simulink model "PID"  (R2021a)
settings: Solver=FixedStepAuto  StartTime=0.0  StopTime=1  FixedStep=0.01  MaxStep=1  RelTol=1e-3
settings Model: Creator=Admin  LastModifiedBy=Admin

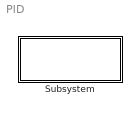
== system PID ==
  Subsystem : Subsystem

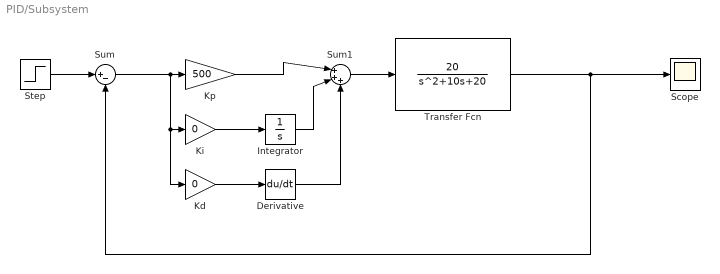
== system PID/Subsystem ==
  Derivative : Derivative
  Integrator : Integrator
  Kd : Gain  Gain=0
  Ki : Gain  Gain=0
  Kp : Gain  Gain=500
  Scope : Scope
  Step : Step  Time=0  SampleTime=0
  Sum : Sum  Inputs=|+-
  Sum1 : Sum  Inputs=|+++
  Transfer Fcn : TransferFcn  Numerator=[20]  Denominator=[1 10 20]
  wires:
  Transfer Fcn/1 -> Sum/2, Scope/1
  Step/1 -> Sum/1
  Sum/1 -> Kd/1, Ki/1, Kp/1
  Ki/1 -> Integrator/1
  Kd/1 -> Derivative/1
  Kp/1 -> Sum1/1
  Sum1/1 -> Transfer Fcn/1
  Integrator/1 -> Sum1/2
  Derivative/1 -> Sum1/3
